simulink model "PMSM_MCBS_Model"  (R2020a)
settings: configuration reference "Sim" (kept outside this file)
PreLoadFcn:
  | % Load modeSchedulerEnum if required
  | if ~exist('modeSchedulerEnum','class')
  |   load_system('ModeLogicModule');
  | end
undefined symbols (not defined in the file): adc, discInertia, encoder, inverter, pmsm, pmsmCoulombFrictionTorque, pmsmInertia, pmsmViscousFrictionCoefficient, pwm, sampleTime
libraries: mcbplantlib x1, autolibpmsmexterior x1
settings Model: DataDictionary=TIKitPlantData.sldd  EnableAccessToBaseWorkspace=off  OrderedModelArguments=off  Creator=promero  LastModifiedBy=RemoteGoat
settings ConfigSetRef: SourceName=Sim

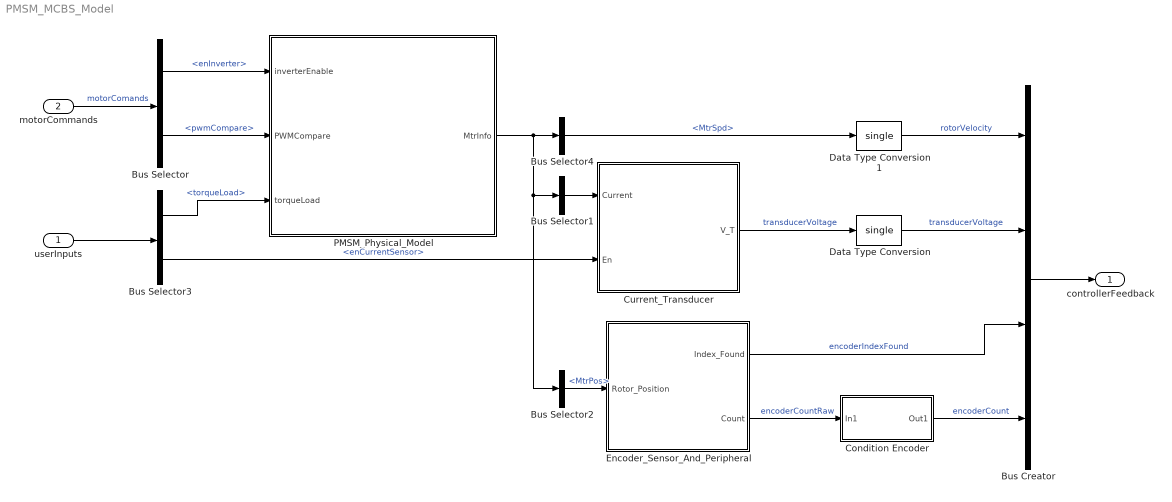
== system PMSM_MCBS_Model ==
  userInputs : Inport  OutDataTypeStr=Bus: userInputs  PortDimensions=1
  motorCommands : Inport  Port=2  OutDataTypeStr=Bus: motorCommands
  Bus Creator : BusCreator  Inputs=4  OutDataTypeStr=Bus: controllerFeedback
      settings: InheritFromInputs=off
  Bus Selector : BusSelector  OutputSignals=enInverter,pwmCompare
  Bus Selector1 : BusSelector  OutputSignals=IaStator,IbStator  OutputAsBus=on
  Bus Selector2 : BusSelector  OutputSignals=MtrPos
  Bus Selector3 : BusSelector  OutputSignals=torqueLoad,enCurrentSensor
  Bus Selector4 : BusSelector  OutputSignals=MtrSpd
  Condition Encoder : Subsystem  mask(Speedgoat Encoder Counter){cntsPerRevolution=encoder.CountPerRevolution, positiveDirection=encoder.ALeadsB}
      mask prompts: cntsPerRevolution "Counts per revolution"; positiveDirection "A leads B?"
      mask help: Configures the direction and positive range of the counter value returned by the Speedgoat IO313 QAD Read block.
      mask init:
      | if positiveDirection == 1
      |     strPositiveDirection = 'A Leads B';
      | else
      |     strPositiveDirection = 'B Leads A';
      | end
      mask Display: fprintf(['Encoder\nPositive Direction:\n' strPositiveDirection]);
  Current_Transducer : Subsystem
      mask Display: image('currentTransducerMask.png');
  Data Type Conversion : DataTypeConversion  OutDataTypeStr=single
  Data Type Conversion1 : DataTypeConversion  OutDataTypeStr=single
  Encoder_Sensor_And_Peripheral : Subsystem
      mask Display:
      | image('encoderSensorAndPeripheralMask.png')
      | port_label('input',1,'P')
      | port_label('output',1,sprintf('Index\nFound'))
      | port_label('output',2,'Count')
  PMSM_Physical_Model : Subsystem
      mask Display: image('focVelocityMotorAndLoadMask.png');
  controllerFeedback : Outport  OutDataTypeStr=Bus: controllerFeedback  VectorParamsAs1DForOutWhenUnconnected=off
  wires:
  Bus Selector3/1 -> PMSM_Physical_Model/3(torqueLoad)  "<torqueLoad>"
  Bus Selector2/1 -> Encoder_Sensor_And_Peripheral/1(Rotor_Position)  "<MtrPos>"
  Bus Selector/2 -> PMSM_Physical_Model/2(PWMCompare)  "<pwmCompare>"
  motorCommands/1 -> Bus Selector/1  "motorComands"
  Encoder_Sensor_And_Peripheral/2(Count) -> Condition Encoder/1(In1)  "encoderCountRaw"
  Encoder_Sensor_And_Peripheral/1(Index_Found) -> Bus Creator/3  "encoderIndexFound"
  Bus Selector3/2 -> Current_Transducer/2(En)  "<enCurrentSensor>"
  Condition Encoder/1(Out1) -> Bus Creator/4  "encoderCount"
  Bus Selector/1 -> PMSM_Physical_Model/1(inverterEnable)  "<enInverter>"
  Bus Selector1/1 -> Current_Transducer/1(Current)
  Current_Transducer/1(V_T) -> Data Type Conversion/1  "transducerVoltage"
  userInputs/1 -> Bus Selector3/1
  Bus Creator/1 -> controllerFeedback/1
  PMSM_Physical_Model/1(MtrInfo) -> Bus Selector2/1, Bus Selector1/1, Bus Selector4/1
  Data Type Conversion/1 -> Bus Creator/2  "transducerVoltage"
  Bus Selector4/1 -> Data Type Conversion1/1  "<MtrSpd>"
  Data Type Conversion1/1 -> Bus Creator/1  "rotorVelocity"

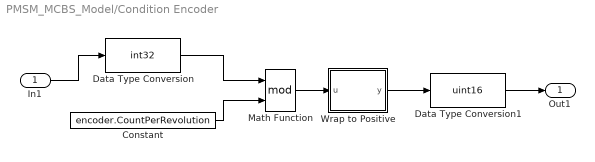
== system PMSM_MCBS_Model/Condition Encoder ==
  In1 : Inport
  Constant : Constant  Value=encoder.CountPerRevolution  OutDataTypeStr=int32
  Data Type Conversion : DataTypeConversion  OutDataTypeStr=int32
  Data Type Conversion1 : DataTypeConversion  OutDataTypeStr=uint16
  Math Function : Math  Operator=mod  SignedPower=on  SaturateOnIntegerOverflow=on
  Wrap to Positive : MATLAB Function  TreatAsAtomicUnit=on
  Out1 : Outport  VectorParamsAs1DForOutWhenUnconnected=off
  wires:
  Math Function/1 -> Wrap to Positive/1(u)
  Constant/1 -> Math Function/2
  In1/1 -> Data Type Conversion/1
  Wrap to Positive/1(y) -> Data Type Conversion1/1
  Data Type Conversion/1 -> Math Function/1
  Data Type Conversion1/1 -> Out1/1

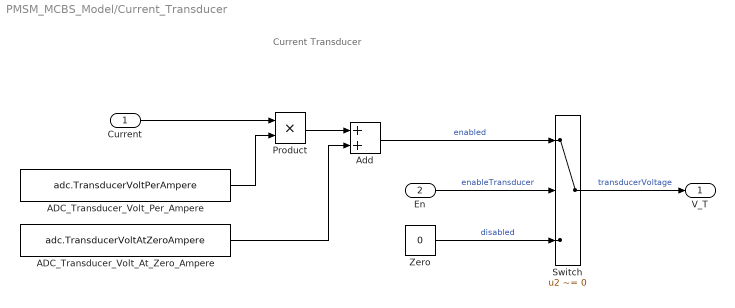
== system PMSM_MCBS_Model/Current_Transducer ==
  note: Current Transducer
  Current : Inport
  En : Inport  Port=2
  ADC_Transducer_Volt_At_Zero_Ampere : Constant  Value=adc.TransducerVoltAtZeroAmpere
  ADC_Transducer_Volt_Per_Ampere : Constant  Value=adc.TransducerVoltPerAmpere
  Add : Sum
  Product : Product  RndMeth=Zero
  Switch : Switch  Criteria=u2 ~= 0
  Zero : Constant  Value=0
  V_T : Outport  VectorParamsAs1DForOutWhenUnconnected=off
  wires:
  Current/1 -> Product/1
  ADC_Transducer_Volt_At_Zero_Ampere/1 -> Add/2
  Product/1 -> Add/1
  ADC_Transducer_Volt_Per_Ampere/1 -> Product/2
  Zero/1 -> Switch/3  "disabled"
  Switch/1 -> V_T/1  "transducerVoltage"
  Add/1 -> Switch/1  "enabled"
  En/1 -> Switch/2  "enableTransducer"

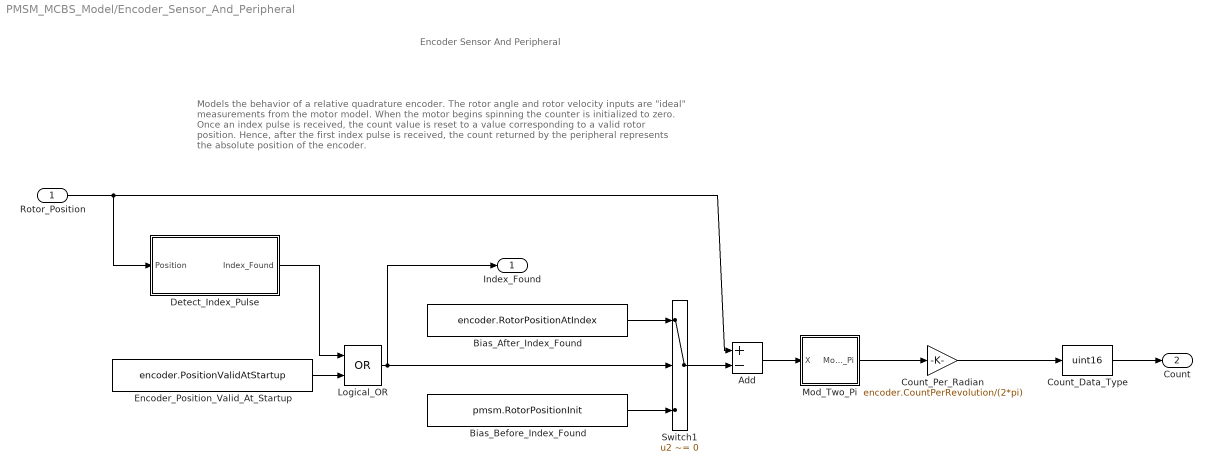
== system PMSM_MCBS_Model/Encoder_Sensor_And_Peripheral ==
  note: Models the behavior of a relative quadrature encoder. The rotor angle and rotor velocity inputs are "ideal" measurements from the motor model.
      | When the motor begins spinning the counter is initialized to zero.
      | Once an index pulse is received, the count value is reset to a value corresponding to a valid rotor position.
      | Hence, after the first index pulse is received, the count returned by the peripheral represents the absolute position of the encoder.
  note: Encoder Sensor And Peripheral
  Rotor_Position : Inport
  Add : Sum  Inputs=+-
  Bias_After_Index_Found : Constant  Value=encoder.RotorPositionAtIndex
  Bias_Before_Index_Found : Constant  Value=pmsm.RotorPositionInit
  Count_Data_Type : DataTypeConversion  OutDataTypeStr=uint16
  Count_Per_Radian : Gain  Gain=encoder.CountPerRevolution/(2*pi)
      settings: AttributesFormatString=|
      | ------------------------------------------
      | Gain = %<Gain>
  Detect_Index_Pulse : Subsystem
  Encoder_Position_Valid_At_Startup : Constant  Value=encoder.PositionValidAtStartup
  Logical_OR : Logic  Operator=OR  IconShape=distinctive  AllPortsSameDT=off  OutDataTypeStr=boolean
  Mod_Two_Pi : Subsystem
      mask Display:
      | text(0.5, 0.5,'Mod 2\pi',...
      |   'HorizontalAlignment', 'Center',...
      |   'VerticalAlignment', 'Middle',...
      |   'texmode', 'on')
  Switch1 : Switch  Criteria=u2 ~= 0
  Index_Found : Outport  VectorParamsAs1DForOutWhenUnconnected=off
  Count : Outport  Port=2  VectorParamsAs1DForOutWhenUnconnected=off
  wires:
  Bias_Before_Index_Found/1 -> Switch1/3
  Bias_After_Index_Found/1 -> Switch1/1
  Logical_OR/1 -> Index_Found/1, Switch1/2
  Encoder_Position_Valid_At_Startup/1 -> Logical_OR/2
  Detect_Index_Pulse/1(Index_Found) -> Logical_OR/1
  Rotor_Position/1 -> Add/1, Detect_Index_Pulse/1(Position)
  Mod_Two_Pi/1(Mod_X_Two_Pi) -> Count_Per_Radian/1
  Count_Data_Type/1 -> Count/1
  Switch1/1 -> Add/2
  Add/1 -> Mod_Two_Pi/1(X)
  Count_Per_Radian/1 -> Count_Data_Type/1

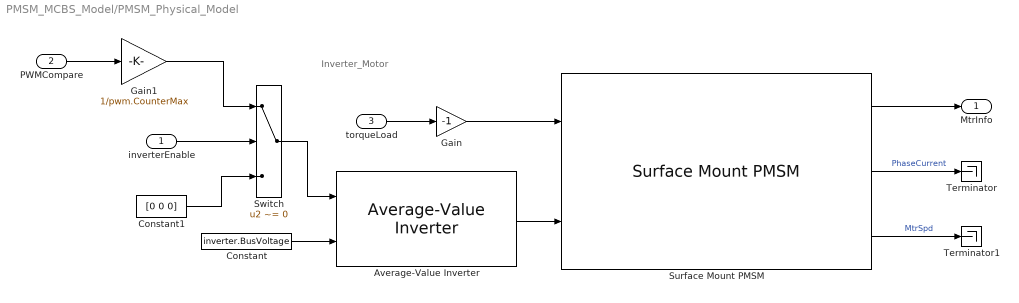
== system PMSM_MCBS_Model/PMSM_Physical_Model ==
  note: Inverter_Motor
  inverterEnable : Inport
  PWMCompare : Inport  Port=2
  torqueLoad : Inport  Port=3
  Average-Value Inverter : mcbplantlib/Average-Value Inverter
  Constant : Constant  Value=inverter.BusVoltage
  Constant1 : Constant  Value=[0 0 0]
  Gain : Gain  Gain=-1
  Gain1 : Gain  Gain=1/pwm.CounterMax
      settings: AttributesFormatString=|
      | ----------------------------------------
      | Gain = %<Gain>
  Surface Mount PMSM : autolibpmsmexterior/Surface Mount PMSM  port_config=Torque  sim_type=Discrete  Ts=sampleTime.CurrentControl  P=pmsm.PolePairs  Rs=pmsm.StatorPhaseResistance  Ldq_=pmsm.InductanceLd  KConstText=Permanent flux linkage constant (lambda_pm):  lambda_pm=pmsm.FluxLinkage  Ke=159.9771  Kt=pmsm.TorqueConstant  mechanical=[pmsmInertia+discInertia, pmsmViscousFrictionCoefficient, pmsmCoulombFrictionTorque]  idq0=[0 0]  theta_init=pmsm.RotorPositionInit - 2*pi  omega_init=pmsm.RotorVelocityInit  KConst=pmsm.FluxLinkage  lambda_pm_calc=pmsm.FluxLinkage  RefBlkName='autolibpmsmexterior/Surface Mount PMSM'  aMode=5  Ldq="[0.0017      0.0017]"
      settings: SourceProductBaseCode=PW,MT,VE,VP
  Switch : Switch  Criteria=u2 ~= 0
  Terminator : Terminator
  Terminator1 : Terminator
  MtrInfo : Outport  VectorParamsAs1DForOutWhenUnconnected=off
  wires:
  PWMCompare/1 -> Gain1/1
  torqueLoad/1 -> Gain/1
  Surface Mount PMSM/1 -> MtrInfo/1
  Switch/1 -> Average-Value Inverter/1
  Constant1/1 -> Switch/3
  inverterEnable/1 -> Switch/2
  Gain/1 -> Surface Mount PMSM/1
  Constant/1 -> Average-Value Inverter/2
  Average-Value Inverter/1 -> Surface Mount PMSM/2
  Gain1/1 -> Switch/1
  Surface Mount PMSM/2 -> Terminator/1  "PhaseCurrent"
  Surface Mount PMSM/3 -> Terminator1/1  "MtrSpd"

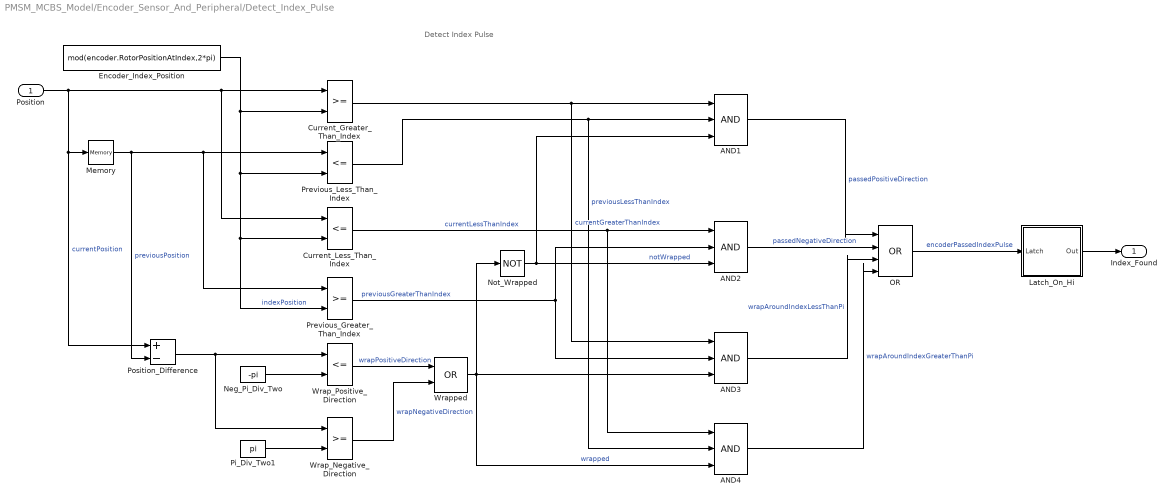
== system PMSM_MCBS_Model/Encoder_Sensor_And_Peripheral/Detect_Index_Pulse ==
  note: Detect Index Pulse
  Position : Inport
  AND{1..4} (4 alike) : Logic  Inputs=3  IconShape=distinctive  AllPortsSameDT=off  OutDataTypeStr=boolean
  Current_Greater_Than_Index : RelationalOperator  OutDataTypeStr=boolean  RndMeth=Nearest
  Current_Less_Than_Index : RelationalOperator  Operator=<=  OutDataTypeStr=boolean  RndMeth=Nearest
  Encoder_Index_Position : Constant  Value=mod(encoder.RotorPositionAtIndex,2*pi)
  Latch_On_Hi : Subsystem
  Memory : Memory  InheritSampleTime=on
  Neg_Pi_Div_Two : Constant  Value=-pi
  Not_Wrapped : Logic  Operator=NOT  IconShape=distinctive  AllPortsSameDT=off  OutDataTypeStr=boolean
  OR : Logic  Operator=OR  Inputs=4  IconShape=distinctive  AllPortsSameDT=off  OutDataTypeStr=boolean
  Pi_Div_Two1 : Constant  Value=pi
  Position_Difference : Sum  Inputs=+-
  Previous_Greater_Than_Index : RelationalOperator  OutDataTypeStr=boolean  RndMeth=Nearest
  Previous_Less_Than_Index : RelationalOperator  Operator=<=  OutDataTypeStr=boolean  RndMeth=Nearest
  Wrap_Negative_Direction : RelationalOperator  OutDataTypeStr=boolean  RndMeth=Nearest
  Wrap_Positive_Direction : RelationalOperator  Operator=<=  OutDataTypeStr=boolean  RndMeth=Nearest
  Wrapped : Logic  Operator=OR  IconShape=distinctive  AllPortsSameDT=off  OutDataTypeStr=boolean
  Index_Found : Outport  VectorParamsAs1DForOutWhenUnconnected=off
  wires:
  AND2/1 -> OR/2  "passedNegativeDirection"
  AND1/1 -> OR/1  "passedPositiveDirection"
  Current_Less_Than_Index/1 -> AND2/1, AND4/1  "currentLessThanIndex"
  Previous_Greater_Than_Index/1 -> AND2/2, AND3/2  "previousGreaterThanIndex"
  OR/1 -> Latch_On_Hi/1(Latch)  "encoderPassedIndexPulse"
  Encoder_Index_Position/1 -> Previous_Less_Than_Index/2, Previous_Greater_Than_Index/2, Current_Less_Than_Index/2, Current_Greater_Than_Index/2  "indexPosition"
  Previous_Less_Than_Index/1 -> AND1/2, AND4/2  "previousLessThanIndex"
  Current_Greater_Than_Index/1 -> AND3/1, AND1/1  "currentGreaterThanIndex"
  Memory/1 -> Position_Difference/2, Previous_Greater_Than_Index/1, Previous_Less_Than_Index/1  "previousPosition"
  Position/1 -> Memory/1, Position_Difference/1, Current_Less_Than_Index/1, Current_Greater_Than_Index/1  "currentPosition"
  Position_Difference/1 -> Wrap_Negative_Direction/1, Wrap_Positive_Direction/1
  Wrap_Positive_Direction/1 -> Wrapped/1  "wrapPositiveDirection"
  Neg_Pi_Div_Two/1 -> Wrap_Positive_Direction/2
  Wrap_Negative_Direction/1 -> Wrapped/2  "wrapNegativeDirection"
  Pi_Div_Two1/1 -> Wrap_Negative_Direction/2
  AND3/1 -> OR/3  "wrapAroundIndexLessThanPi"
  Latch_On_Hi/1(Out) -> Index_Found/1
  Not_Wrapped/1 -> AND1/3, AND2/3  "notWrapped"
  Wrapped/1 -> AND4/3, AND3/3, Not_Wrapped/1  "wrapped"
  AND4/1 -> OR/4  "wrapAroundIndexGreaterThanPi"

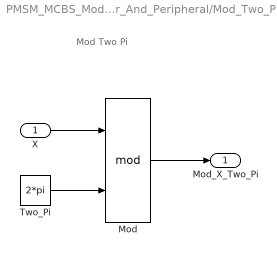
== system PMSM_MCBS_Model/Encoder_Sensor_And_Peripheral/Mod_Two_Pi ==
  note: Mod Two Pi
  X : Inport
  Mod : Math  Operator=mod  SignedPower=on  SaturateOnIntegerOverflow=on
  Two_Pi : Constant  Value=2*pi  OutDataTypeStr=Inherit: Inherit via back propagation
  Mod_X_Two_Pi : Outport  VectorParamsAs1DForOutWhenUnconnected=off
  wires:
  X/1 -> Mod/1
  Two_Pi/1 -> Mod/2
  Mod/1 -> Mod_X_Two_Pi/1

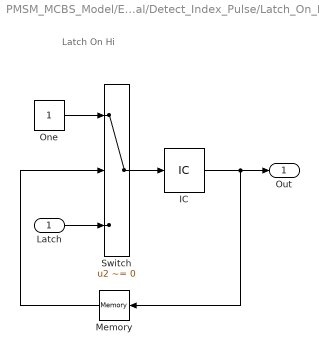
== system PMSM_MCBS_Model/Encoder_Sensor_And_Peripheral/Detect_Index_Pulse/Latch_On_Hi ==
  note: Latch On Hi
  Latch : Inport
  IC : InitialCondition  Value=0
  Memory : Memory  InheritSampleTime=on
  One : Constant  OutDataTypeStr=boolean
  Switch : Switch  Criteria=u2 ~= 0  Threshold=1
  Out : Outport  VectorParamsAs1DForOutWhenUnconnected=off
  wires:
  IC/1 -> Memory/1, Out/1
  Latch/1 -> Switch/3
  Switch/1 -> IC/1
  One/1 -> Switch/1
  Memory/1 -> Switch/2

== matlab function PMSM_MCBS_Model/Condition Encoder/Wrap to Positive ==
  data: u input; y output; cntsPerRevolution parameter; positiveDirection parameter
function y = fcn(u,cntsPerRevolution,positiveDirection)
% Guarantee the count is between 0 and cntsPerRevolution
% (Speedgoat count can be negative)

% Simplest case
y=u;

% % Max consecutive index pulses that can be missed
% maxIndexPulseMissesToRecoverFrom = 2;
% 
% for index = 1:maxIndexPulseMissesToRecoverFrom
%     if y >= cntsPerRevolution
%         y = y - cntsPerRevolution;
%     elseif y < -cntsPerRevolution
%         y = y + cntsPerRevolution;
%     end
% end
% 
% % Wrap angle to positive value
% if (y<0)
%     y = cntsPerRevolution + y;
% end

% Handle case of swapping encoder A & B signals
if positiveDirection ~= 1
    y = (cntsPerRevolution-1) - y;
end
